simulink model "chuas_control"  (R2016b)
settings: Solver=VariableStepAuto  StartTime=0.0  StopTime=10.0  RelTol=1e-3
values from neighbouring files (symbols this model uses):
  A = [-18/7 9 0;1 -1 1;0 -14.28 0]    [chuas.m]
  H = [27/7;0;0]    [chuas.m]
  K = inv(Ph)*Vh    [chuas.m]
settings Model: Creator=A  LastModifiedBy=yeyuhang
settings DataIOCC: ReturnWorkspaceOutputs=on
settings SFSimCC: SimUseLocalCustomCode=on
settings RTWCC: RTWUseLocalCustomCode=on

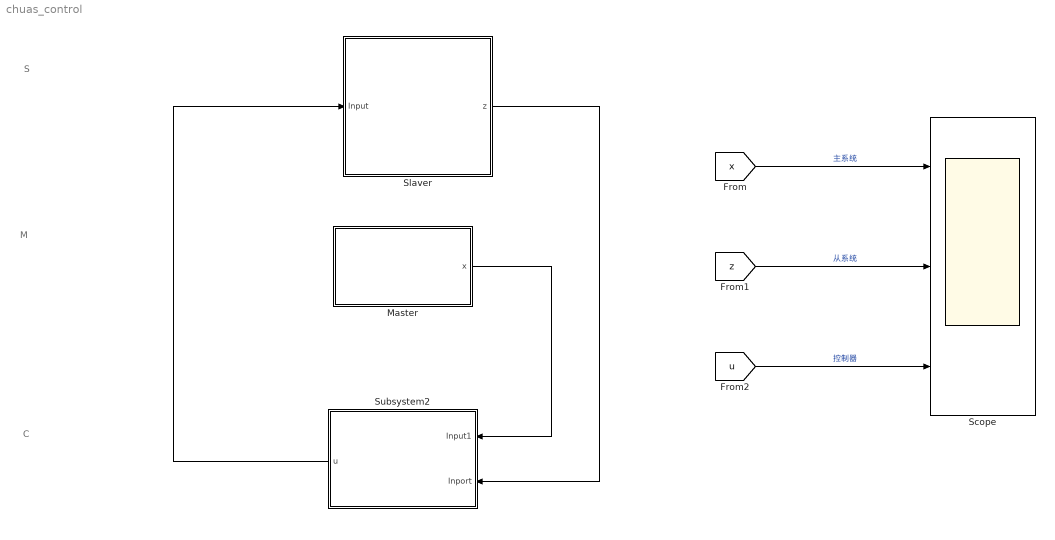
== system chuas_control ==
  note: M
  note: S
  note: C
  Master : Subsystem
  Scope : Scope  NumInputPorts=3
  Slaver : Subsystem
  Subsystem2 : Subsystem
  wires:
  Subsystem2/1(u) -> Slaver/1(Input)
  Master/1(x) -> Subsystem2/1(Input1)
  Slaver/1(z) -> Subsystem2/2(Inport)
  [z] -> Scope/2  "从系统"
  [u] -> Scope/3  "控制器"
  [x] -> Scope/1  "主系统"

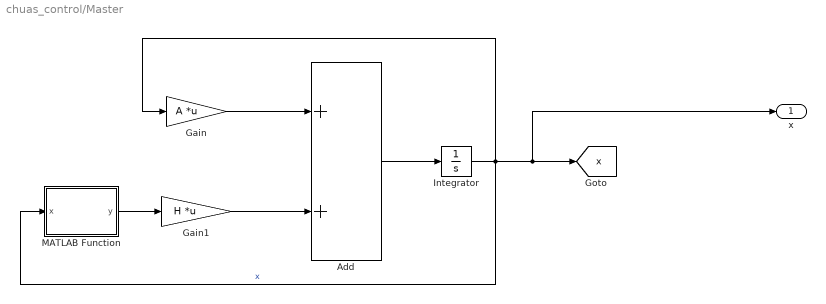
== system chuas_control/Master ==
  Add : Sum
  Gain : Gain  Gain=A  Multiplication=Matrix(K*u)
  Gain1 : Gain  Gain=H  Multiplication=Matrix(K*u)
  Integrator : Integrator  InitialCondition=[0.1 0.2 0.3]
  MATLAB Function : MATLAB Function  TreatAsAtomicUnit=on
  x : Outport
  tag scope: x=global
  wires:
  Integrator/1 -> Gain/1, MATLAB Function/1(x), x/1, [x]  "x"
  Gain1/1 -> Add/2
  MATLAB Function/1(y) -> Gain1/1
  Add/1 -> Integrator/1
  Gain/1 -> Add/1

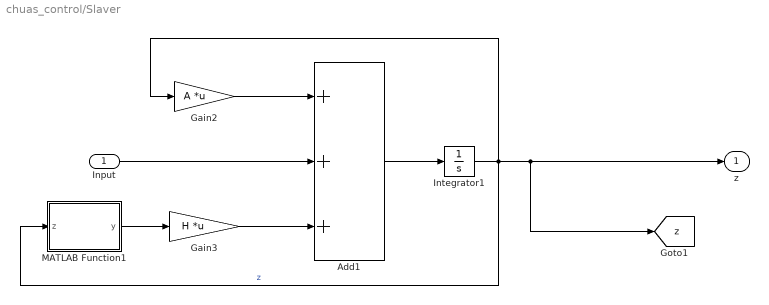
== system chuas_control/Slaver ==
  Input : Inport
  Add1 : Sum  Inputs=+++
  Gain2 : Gain  Gain=A  Multiplication=Matrix(K*u)
  Gain3 : Gain  Gain=H  Multiplication=Matrix(K*u)
  Integrator1 : Integrator  InitialCondition=[1 2 3]
  MATLAB Function1 : MATLAB Function  TreatAsAtomicUnit=on
  z : Outport
  tag scope: z=global
  wires:
  Gain2/1 -> Add1/1
  Integrator1/1 -> Gain2/1, MATLAB Function1/1(z), z/1, [z]  "z"
  Input/1 -> Add1/2
  Gain3/1 -> Add1/3
  MATLAB Function1/1(y) -> Gain3/1
  Add1/1 -> Integrator1/1

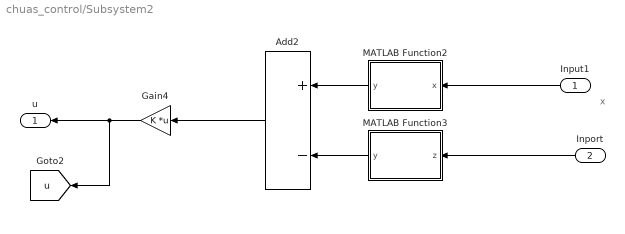
== system chuas_control/Subsystem2 ==
  note: x
  Input1 : Inport
  Inport : Inport  Port=2
  Add2 : Sum  Inputs=+-
  Gain4 : Gain  Gain=K  Multiplication=Matrix(K*u)
  MATLAB Function2 : MATLAB Function  TreatAsAtomicUnit=on
  MATLAB Function3 : MATLAB Function  TreatAsAtomicUnit=on
  u : Outport
  tag scope: u=global
  wires:
  Gain4/1 -> u/1, [u]
  MATLAB Function3/1(y) -> Add2/2
  Input1/1 -> MATLAB Function2/1(x)
  Add2/1 -> Gain4/1
  Inport/1 -> MATLAB Function3/1(z)
  MATLAB Function2/1(y) -> Add2/1

== matlab function chuas_control/Slaver/MATLAB Function1 ==
  data: z input; y output
function y = fcn(z)
C=[1 0 0];
y =(1/2)*(abs(C*z+1)-abs(C*z-1));

== matlab function chuas_control/Subsystem2/MATLAB Function2 ==
  data: x input; y output
function y = fcn(x)
C=[1,0,0];
y =C*x;

== matlab function chuas_control/Subsystem2/MATLAB Function3 ==
  data: z input; y output
function y = fcn(z)
C=[1,0,0];

y = C*z;

== matlab function chuas_control/Master/MATLAB Function ==
  data: x input; y output
function y = fcn(x)

C=[1 0 0];
y =(1/2)*(abs(C*x+1)-abs(C*x-1));
